simulink model "OmnidirectionalVehicle"  (R2016b)
settings: Solver=FixedStepAuto  StartTime=0.0  StopTime=inf  FixedStep=0.01  RelTol=1e-3
PreLoadFcn:
  | addpath('solvetime');
libraries: simulink x5
settings Model: Creator=gaoweijin  LastModifiedBy=gaoweijin

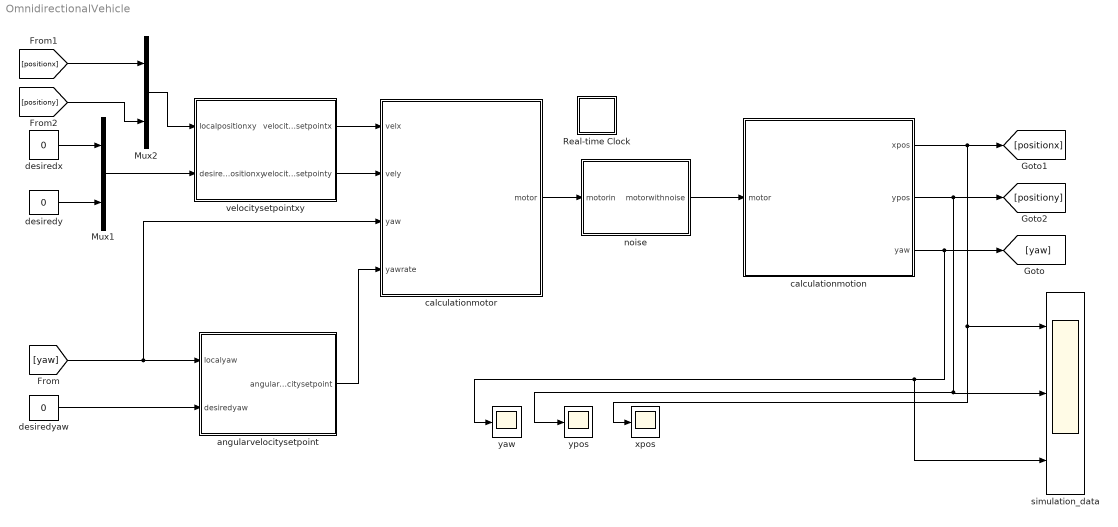
== system OmnidirectionalVehicle ==
  Mux1 : Mux  Inputs=2
  Mux2 : Mux  Inputs=2
  Real-time Clock : Subsystem  mask(Real-time Clock){sample_time=0.01, tolerance=1}
      mask prompts: sample_time "Synchronize with real-time every n seconds:"; tolerance "Real-time warning tolerance (seconds):"
      mask help: Real-time Synchronization Block
      mask Help: This block synchronizes simulation time with the PC real-time clock or UNIX system clock. The first dialog entry is the period at which the clock is checked to insure real-time synchronization. The second dialog entry is the number of seconds that the simulation time must be within real-time before a warning is printed.
      mask Display: plot(0,0,100,100,[40,60,60,54,54,64,69,76,82,77,81,83,83,81,78,74,70,64,57,49,41,35,32,30,30,31,34,40,47,47,40,40],[90,90,85,85,80,79,76,87,80,70,64,57,49,41,33,28,24,22,21,23,25,31,37,46,56,65,73,78,80,85,85,90],[69,53,53],[64,50,73])
  angularvelocitysetpoint : Subsystem
  calculationmotion : Subsystem
  calculationmotor : Subsystem
  desiredx : Constant  Value=0
  desiredy : Constant  Value=0
  desiredyaw : Constant  Value=0
  noise : Subsystem
  simulation_data : Scope  NumInputPorts=3
  velocitysetpointxy : Subsystem
  xpos : Scope
  yaw : Scope
  ypos : Scope
  wires:
  desiredx/1 -> Mux1/1
  desiredy/1 -> Mux1/2
  Mux1/1 -> velocitysetpointxy/2(desiredpositionxy)
  desiredyaw/1 -> angularvelocitysetpoint/2(desiredyaw)
  calculationmotor/1(motor) -> noise/1(motorin)
  noise/1(motorwithnoise) -> calculationmotion/1(motor)
  calculationmotion/2(ypos) -> [positiony], simulation_data/2, ypos/1
  velocitysetpointxy/1(velocitysetpointx) -> calculationmotor/1(velx)
  velocitysetpointxy/2(velocitysetpointy) -> calculationmotor/2(vely)
  calculationmotion/1(xpos) -> xpos/1, simulation_data/1, [positionx]
  calculationmotion/3(yaw) -> [yaw], simulation_data/3, yaw/1
  [yaw] -> calculationmotor/3(yaw), angularvelocitysetpoint/1(localyaw)
  angularvelocitysetpoint/1(angularvelocitysetpoint) -> calculationmotor/4(yawrate)
  [positionx] -> Mux2/1
  Mux2/1 -> velocitysetpointxy/1(localpositionxy)
  [positiony] -> Mux2/2

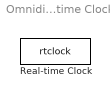
== system OmnidirectionalVehicle/Real-time Clock ==
  Real-time Clock : S-Function  FunctionName=rtclock  Parameters=sample_time, tolerance  SFunctionDeploymentMode=off  EnableBusSupport=off

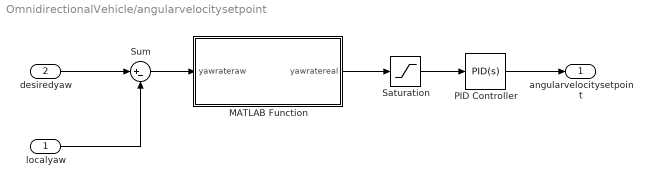
== system OmnidirectionalVehicle/angularvelocitysetpoint ==
  localyaw : Inport
  desiredyaw : Inport  Port=2
  MATLAB Function : MATLAB Function  TreatAsAtomicUnit=on
  PID Controller : simulink/Continuous/PID Controller  Controller=PID  TimeDomain=Continuous-time  SampleTime=-1  IntegratorMethod=Forward Euler  FilterMethod=Forward Euler  Form=Parallel  UseFilter=on  ControllerParametersSource=internal  P=16  I=0  D=0.2  N=100  InitialConditionSource=internal  InitialConditionForIntegrator=0  InitialConditionForFilter=0  ExternalReset=none  LimitOutput=off  UpperSaturationLimit=inf  LowerSaturationLimit=-inf  LinearizeAsGain=on  AntiWindupMode=none  Kb=1  TrackingMode=off  Kt=1  PParamMin=[]  PParamMax=[]  IParamMin=[]  IParamMax=[]  DParamMin=[]  DParamMax=[]  NParamMin=[]  NParamMax=[]  KbParamMin=[]  KbParamMax=[]  KtParamMin=[]  KtParamMax=[]  POutMin=[]  POutMax=[]  IOutMin=[]  IOutMax=[]  DOutMin=[]  DOutMax=[]  NOutMin=[]  NOutMax=[]  KbOutMin=[]  KbOutMax=[]  KtOutMin=[]  KtOutMax=[]  IntegratorOutMin=[]  IntegratorOutMax=[]  FilterOutMin=[]  FilterOutMax=[]  SumOutMin=[]  SumOutMax=[]  SumI1OutMin=[]  SumI1OutMax=[]  SumI2OutMin=[]  SumI2OutMax=[]  SumI3OutMin=[]  SumI3OutMax=[]  SumDOutMin=[]  SumDOutMax=[]  SaturationOutMin=[]  SaturationOutMax=[]  IntegratorContinuousStateAttributes=''  IntegratorStateMustResolveToSignalObject=off  IntegratorRTWStateStorageClass=Auto  FilterContinuousStateAttributes=''  FilterStateMustResolveToSignalObject=off  FilterRTWStateStorageClass=Auto  DifferentiatorICPrevScaledInput=0  DifferentiatorOutMin=[]  DifferentiatorOutMax=[]
  Saturation : Saturate  UpperLimit=45  LowerLimit=-45
  Sum : Sum  Inputs=|+-
  angularvelocitysetpoint : Outport
  wires:
  PID Controller/1 -> angularvelocitysetpoint/1
  Sum/1 -> MATLAB Function/1(yawrateraw)
  MATLAB Function/1(yawratereal) -> Saturation/1
  Saturation/1 -> PID Controller/1
  localyaw/1 -> Sum/2
  desiredyaw/1 -> Sum/1

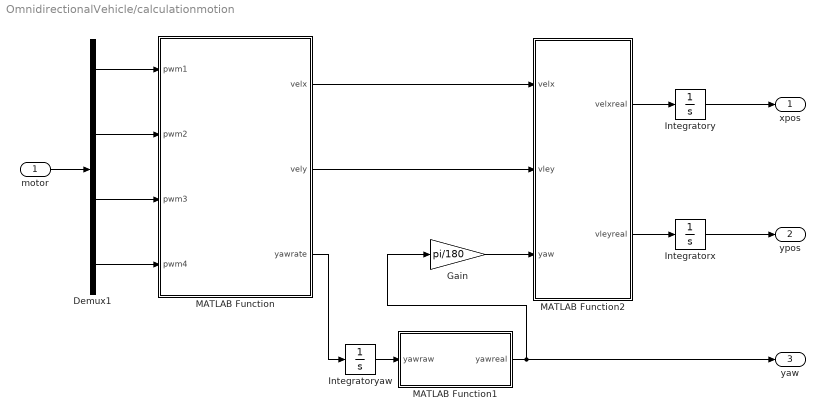
== system OmnidirectionalVehicle/calculationmotion ==
  motor : Inport
  Demux1 : Demux
  Gain : Gain  Gain=pi/180
  Integratorx : Integrator
  Integratory : Integrator
  Integratoryaw : Integrator
  MATLAB Function : MATLAB Function  TreatAsAtomicUnit=on
  MATLAB Function1 : MATLAB Function  TreatAsAtomicUnit=on
  MATLAB Function2 : MATLAB Function  TreatAsAtomicUnit=on
  xpos : Outport
  ypos : Outport  Port=2
  yaw : Outport  Port=3
  wires:
  MATLAB Function/3(yawrate) -> Integratoryaw/1
  Demux1/1 -> MATLAB Function/1(pwm1)
  Demux1/2 -> MATLAB Function/2(pwm2)
  Demux1/3 -> MATLAB Function/3(pwm3)
  Demux1/4 -> MATLAB Function/4(pwm4)
  motor/1 -> Demux1/1
  Integratoryaw/1 -> MATLAB Function1/1(yawraw)
  MATLAB Function1/1(yawreal) -> yaw/1, Gain/1
  Gain/1 -> MATLAB Function2/3(yaw)
  MATLAB Function/1(velx) -> MATLAB Function2/1(velx)
  MATLAB Function2/1(velxreal) -> Integratory/1
  Integratory/1 -> xpos/1
  MATLAB Function2/2(vleyreal) -> Integratorx/1
  Integratorx/1 -> ypos/1
  MATLAB Function/2(vely) -> MATLAB Function2/2(vley)

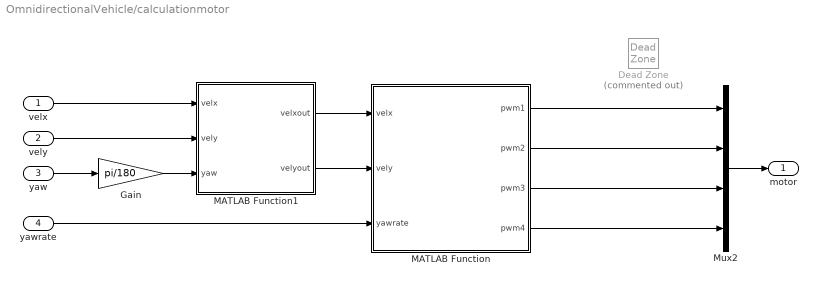
== system OmnidirectionalVehicle/calculationmotor ==
  velx : Inport
  vely : Inport  Port=2
  yaw : Inport  Port=3
  yawrate : Inport  Port=4
  Dead Zone : DeadZone  Commented=on  LowerValue=-0.05  UpperValue=0.05  SaturateOnIntegerOverflow=on
  Gain : Gain  Gain=pi/180
  MATLAB Function : MATLAB Function  TreatAsAtomicUnit=on
  MATLAB Function1 : MATLAB Function  TreatAsAtomicUnit=on
  Mux2 : Mux
  motor : Outport
  wires:
  yawrate/1 -> MATLAB Function/3(yawrate)
  Mux2/1 -> motor/1
  MATLAB Function/1(pwm1) -> Mux2/1
  MATLAB Function/2(pwm2) -> Mux2/2
  MATLAB Function/3(pwm3) -> Mux2/3
  MATLAB Function/4(pwm4) -> Mux2/4
  MATLAB Function1/1(velxout) -> MATLAB Function/1(velx)
  MATLAB Function1/2(velyout) -> MATLAB Function/2(vely)
  velx/1 -> MATLAB Function1/1(velx)
  vely/1 -> MATLAB Function1/2(vely)
  Gain/1 -> MATLAB Function1/3(yaw)
  yaw/1 -> Gain/1

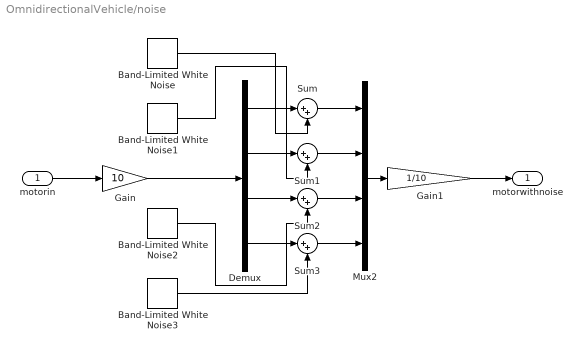
== system OmnidirectionalVehicle/noise ==
  motorin : Inport
  Band-Limited White Noise : simulink/Sources/Band-Limited White Noise  Cov=[0.00001]  Ts=0.1  seed=[23341]
  Band-Limited White Noise1 : simulink/Sources/Band-Limited White Noise  Cov=[0.00001]  Ts=0.1  seed=[23342]
  Band-Limited White Noise2 : simulink/Sources/Band-Limited White Noise  Cov=[0.00001]  Ts=0.1  seed=[23343]
  Band-Limited White Noise3 : simulink/Sources/Band-Limited White Noise  Cov=[0.00001]  Ts=0.1  seed=[23344]
  Demux : Demux
  Gain : Gain  Gain=10
  Gain1 : Gain  Gain=1/10
  Mux2 : Mux
  Sum{,1..3} (4 alike) : Sum  Inputs=|++
  motorwithnoise : Outport
  wires:
  Demux/4 -> Sum3/1
  Band-Limited White Noise/1 -> Sum/2
  Demux/1 -> Sum/1
  Sum/1 -> Mux2/1
  motorin/1 -> Gain/1
  Sum2/1 -> Mux2/3
  Demux/3 -> Sum2/1
  Demux/2 -> Sum1/1
  Sum3/1 -> Mux2/4
  Sum1/1 -> Mux2/2
  Band-Limited White Noise1/1 -> Sum1/2
  Band-Limited White Noise2/1 -> Sum2/2
  Band-Limited White Noise3/1 -> Sum3/2
  Gain/1 -> Demux/1
  Gain1/1 -> motorwithnoise/1
  Mux2/1 -> Gain1/1

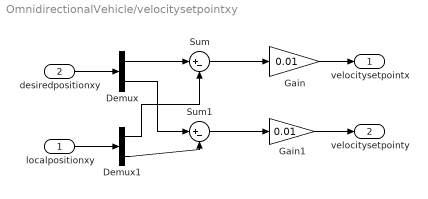
== system OmnidirectionalVehicle/velocitysetpointxy ==
  localpositionxy : Inport
  desiredpositionxy : Inport  Port=2
  Demux : Demux  Outputs=2
  Demux1 : Demux  Outputs=2
  Gain : Gain  Gain=0.01
  Gain1 : Gain  Gain=0.01
  Sum : Sum  Inputs=|+-
  Sum1 : Sum  Inputs=|+-
  velocitysetpointx : Outport
  velocitysetpointy : Outport  Port=2
  wires:
  Gain1/1 -> velocitysetpointy/1
  Gain/1 -> velocitysetpointx/1
  Demux/1 -> Sum/1
  Demux/2 -> Sum1/1
  Demux1/1 -> Sum/2
  Demux1/2 -> Sum1/2
  Sum/1 -> Gain/1
  Sum1/1 -> Gain1/1
  desiredpositionxy/1 -> Demux/1
  localpositionxy/1 -> Demux1/1

== matlab function OmnidirectionalVehicle/calculationmotor/MATLAB Function1 ==
  data: velx input; velxout output; vely input; yaw input; velyout output
function [velxout,velyout] = fcn(velx,vely,yaw)
velxout =  velx*cos(yaw) + vely *sin(yaw);
velyout = -velx*sin(yaw) + vely *cos(yaw);
% velxout = velx;
% velyout = vely;
% velxout =  velx*cos(yaw) - vely *sin(yaw);   %-+ --  +-
% velyout =  velx*sin(yaw) + vely *cos(yaw);

== matlab function OmnidirectionalVehicle/calculationmotor/MATLAB Function ==
  data: velx input; vely input; pwm1 output; yawrate input; pwm2 output; pwm3 output; pwm4 output
function [pwm1,pwm2,pwm3,pwm4]= calculationmotor(velx,vely,yawrate)
L1 = 0.75;
L2 = 0.75;
R = 0.15;
pwm1 = ( velx + vely + (L1+L2)*yawrate)/R;
pwm2 = ( velx - vely - (L1+L2)*yawrate)/R;
pwm3 = ( velx - vely + (L1+L2)*yawrate)/R;
pwm4 = ( velx + vely - (L1+L2)*yawrate)/R;
if pwm1 > 100
  pwm1 = 100;
end
if pwm2 > 100
  pwm2 = 100;
end
if pwm3 > 100
  pwm3 = 100;
end
if pwm4 > 100
  pwm4 = 100;
end
if pwm1 < -100
  pwm1 = -100;
end
if pwm2 < -100
  pwm2 = -100;
end
if pwm3 < -100
  pwm3 = -100;
end
if pwm4 < -100
  pwm4 = -100;
end

== matlab function OmnidirectionalVehicle/calculationmotion/MATLAB Function ==
  data: pwm1 input; velx output; vely output; yawrate output; pwm2 input; pwm3 input; pwm4 input
function [velx,vely,yawrate] = calculationmotion(pwm1,pwm2,pwm3,pwm4)
L1 = 100;
L2 = 100;
R = 20;
velx = (pwm1 + pwm2 + pwm3 +pwm4)*R/4;
vely = (pwm1 - pwm2 - pwm3 +pwm4)*R/4;
tempmiddle = 1/(L1+L2);
yawrate = ( tempmiddle*pwm1 - tempmiddle*pwm2 + tempmiddle*pwm3 - tempmiddle*pwm4)*R/4;

% function velocitysetpointxy = calculationvelocity(localpositionxy,desiredpositionxy)
% tempvel = zeros(2,1);
% tempvel(1) = desiredpositionxy(1)-localpositionxy(1);
% tempvel(2) = desiredpositionxy(2)-localpositionxy(2);
% velocitysetpointxy = tempvel;

== matlab function OmnidirectionalVehicle/calculationmotion/MATLAB Function1 ==
  data: yawraw input; yawreal output
function yawreal = fcn(yawraw)
while yawraw > 180
    yawraw = yawraw -360;
end
while yawraw < -180
    yawraw = yawraw +360;
end
yawreal = yawraw;

== matlab function OmnidirectionalVehicle/angularvelocitysetpoint/MATLAB Function ==
  data: yawrateraw input; yawratereal output
function yawratereal = yawtranslate(yawrateraw)
%正北为x轴，正东为y轴，北偏东为正，北偏西为负。
tempangle = yawrateraw;
if tempangle>180
    tempangle = tempangle - 360;
end 
if tempangle<-180
    tempangle = tempangle + 360;
end

yawratereal = tempangle;

== matlab function OmnidirectionalVehicle/calculationmotion/MATLAB Function2 ==
  data: velx input; velxreal output; vley input; yaw input; vleyreal output
function [velxreal,vleyreal] = fcn(velx,vley,yaw)
velxreal = velx * cos(yaw) - vley * sin(yaw);
vleyreal = velx * sin(yaw) + vley * cos(yaw);
